simulink model "PD_sine_wave_input_final"  (R2022a)
settings: Solver=VariableStepAuto  StartTime=0.0  StopTime=10.0  RelTol=1e-3
libraries: slpidlib x1
settings Model: Creator=Electronica Care  LastModifiedBy=Electronica Care

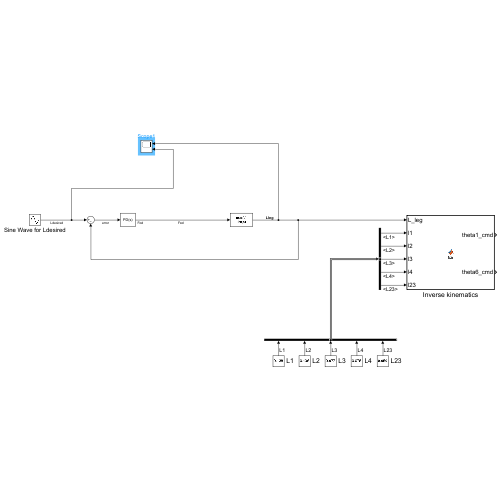
[thumbnail: Simulink's stored preview of the top-level diagram]
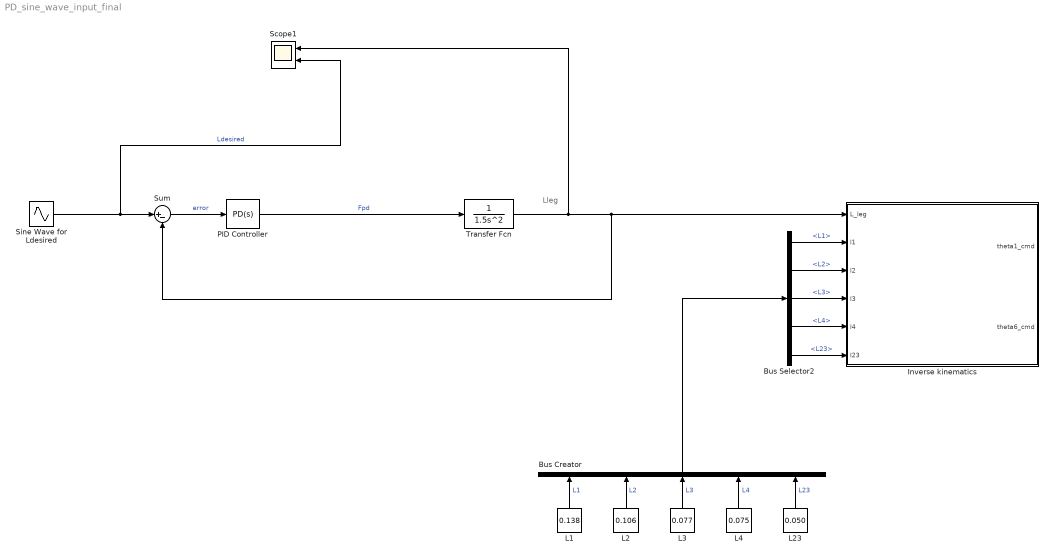
== system PD_sine_wave_input_final ==
  note: Lleg
  Bus Creator : BusCreator  Inputs=5
  Bus Selector2 : BusSelector  OutputSignals=L1,L2,L3,L4,L23
  Inverse kinematics : MATLAB Function  TreatAsAtomicUnit=on
  L1 : Constant  Value=0.138
  L2 : Constant  Value=0.106
  L23 : Constant  Value=0.050
  L3 : Constant  Value=0.077
  L4 : Constant  Value=0.075
  PID Controller : slpidlib/PID Controller  Controller=PD  Form=Parallel  TimeDomain=Continuous-time  UseExternalTs=off  SampleTime=-1  IntegratorMethod=Forward Euler  FilterMethod=Forward Euler  ControllerParametersSource=internal  P=26.8179122674838  I=200  UseKiTs=off  D=14.7354369140272  N=1142.8279760416  UseFilter=on  TunerSelectOption=Transfer Function Based (PID Tuner App)  InitialConditionSource=internal  InitialConditionForIntegrator=0  InitialConditionForFilter=0  DifferentiatorICPrevScaledInput=0  ExternalReset=none  TrackingMode=off  Kt=1  LimitOutput=off  SatLimitsSource=internal  UpperSaturationLimit=inf  LowerSaturationLimit=-inf  LinearizeAsGain=on  AntiWindupMode=none  Kb=1  POutMin=[]  POutMax=[]  IOutMin=[]  IOutMax=[]  DOutMin=[]  DOutMax=[]  NOutMin=[]  NOutMax=[]  SumOutMin=[]  SumOutMax=[]  SaturationOutMin=[]  SaturationOutMax=[]  PParamMin=[]  PParamMax=[]  IParamMin=[]  IParamMax=[]  DParamMin=[]  DParamMax=[]  NParamMin=[]  NParamMax=[]  KbParamMin=[]  KbParamMax=[]  KtParamMin=[]  KtParamMax=[]  KbOutMin=[]  KbOutMax=[]  KtOutMin=[]  KtOutMax=[]  IntegratorOutMin=[]  IntegratorOutMax=[]  FilterOutMin=[]  FilterOutMax=[]  SumI1OutMin=[]  SumI1OutMax=[]  SumI2OutMin=[]  SumI2OutMax=[]  SumI3OutMin=[]  SumI3OutMax=[]  SumI4OutMin=[]  SumI4OutMax=[]  SumDOutMin=[]  SumDOutMax=[]  DifferentiatorOutMin=[]  DifferentiatorOutMax=[]  FilterDiffOutCoefMin=[]  FilterDiffOutCoefMax=[]  ReciprocalOutMin=[]  ReciprocalOutMax=[]  SumDenOutMin=[]  SumDenOutMax=[]  SumNumOutMin=[]  SumNumOutMax=[]  DivideOutMin=[]  DivideOutMax=[]  UdiffTsProdOutMin=[]  UdiffTsProdOutMax=[]  NTsProdOutMin=[]  NTsProdOutMax=[]  UintegralTsProdOutMin=[]  UintegralTsProdOutMax=[]  UngainTsProdOutMin=[]  UngainTsProdOutMax=[]  IntegratorContinuousStateAttributes=''  IntegratorStateMustResolveToSignalObject=off  IntegratorRTWStateStorageClass=Auto  FilterContinuousStateAttributes=''  FilterStateMustResolveToSignalObject=off  FilterRTWStateStorageClass=Auto  ParallelPVariant=InternalParameters  IdealPVariant=Disabled  IVariant=Disabled  DVariant=InternalParameters  IntegratorVariant=Disabled  SatVariant=Disabled  AWVariant=Disabled  PCopyVariant=Disabled  TRVariant=Disabled  FdbkBlocksVariant=Forward  IdealPFdbkVariant=Disabled  SatFdbkVariant=Disabled  DerivativeFilterVariant=ContFilter  NVariant=InternalParameters  NCopyVariant=Disabled  FilterICVariant=InternalICsFilter  IntegratorICVariant=Disabled  ExternalResetVariant=Disabled  TRSumVariant=Passthrough  SumFdbkVariant=Disabled  SumVariant=Sum_PD  TsampFilterVariant=InternalTs  TsampNgainVariant=Passthrough  TsampIntegralVariant=Disabled_SignalSpec  ExternalSaturationOutDataTypeStr=Inherit: Same as second input  aMode=0
  Scope1 : Scope  NumInputPorts=2
  Sine Wave for Ldesired : Sin  Amplitude=0.02  Bias=0.15  Frequency=3.14  SampleTime=0
  Sum : Sum  Inputs=|+-
  Transfer Fcn : TransferFcn  Denominator=[1.5 0 0]
  wires:
  Sum/1 -> PID Controller/1  "error"
  Sine Wave for Ldesired/1 -> Scope1/2, Sum/1  "Ldesired"
  PID Controller/1 -> Transfer Fcn/1  "Fpd"
  Bus Creator/1 -> Bus Selector2/1
  Transfer Fcn/1 -> Scope1/1, Inverse kinematics/1(L_leg), Sum/2
  Bus Selector2/4 -> Inverse kinematics/5(l4)  "<L4>"
  Bus Selector2/2 -> Inverse kinematics/3(l2)  "<L2>"
  Bus Selector2/5 -> Inverse kinematics/6(l23)  "<L23>"
  Bus Selector2/3 -> Inverse kinematics/4(l3)  "<L3>"
  Bus Selector2/1 -> Inverse kinematics/2(l1)  "<L1>"
  L23/1 -> Bus Creator/5  "L23"
  L4/1 -> Bus Creator/4  "L4"
  L2/1 -> Bus Creator/2  "L2"
  L3/1 -> Bus Creator/3  "L3"
  L1/1 -> Bus Creator/1  "L1"

== matlab function PD_sine_wave_input_final/Inverse kinematics ==
  data: L_leg input; theta1_cmd output; l1 input; l2 input; l3 input; l4 input; l23 input; theta6_cmd output
function [theta1_cmd, theta6_cmd] = fcn(L_leg, l1, l2, l3, l4, l23)
    
    arg1 = (L_leg^2 + l2^2 - l1^2) / (2 * L_leg * l2);
    arg1 = max(min(arg1, 1), -1);
    theta1_cmd = asin(arg1);
    
    
    l5 = sqrt(l2^2 + l4^2 - 2*l2*l4*cos(theta1_cmd + pi/4));
    
    
    theta2 = asin((l4 * sin(theta1_cmd + pi/4)) / l5);
    
    
    arg3 = (l23^2 + l5^2 - l3^2) / (2 * l23 * l5);
    arg3 = max(min(arg3, 1), -1);
    theta3 = acos(arg3);
    
    
    theta4 = pi - theta1_cmd - theta2 - theta3;
    
    
    arg6 = (l5 * sin(theta3)) / l3;
    arg6 = max(min(arg6, 1), -1);
    theta6_cmd = asin(arg6) - theta4;
end
